simulink model "parallelParking"  (R2016b)
settings: Solver=FixedStepDiscrete  StartTime=0  StopTime=40  FixedStep=0.1  RelTol=1e-3  EnableMultiTasking=on
model workspace (MAT data in the model file):
  LANE_WIDTH = 0.5
  WORLD_SIZE = Simulink.Parameter
  WORLD_SIZE.Value = 5
  WORLD_SIZE.DataType = 'auto'
  WORLD_SIZE.Dimensions = [1 1]
  dt = Simulink.Parameter
  dt.Value = 0.05
  dt.DataType = 'auto'
  dt.Dimensions = [1 1]
values from neighbouring files (symbols this model uses):
  WORLD_SIZE = 5    [simulation.m]    (also in stateflowSim.m)
settings Model: Creator=larry  LastModifiedBy=larry
settings SolverCC: AutoInsertRateTranBlk=on
settings DataIOCC: LimitDataPoints=on
settings OptimizationCC: LifeSpan=inf
settings DebuggingCC: AllowSymbolicDim=off  SFUnexpectedBacktrackingDiag=warning  SFNoUnconditionalDefaultTransitionDiag=warning  SFExecutionAtInitializationDiag=none
settings GRTTargetCC: TargetLangStandard=C89/C90 (ANSI)  GeneratePreprocessorConditionals=Disable all
settings ConfigComp: CovMetricSettings=dw  CovHtmlReporting=on  CovSaveCumulativeToWorkspaceVar=on  CovSaveSingleToWorkspaceVar=on  CovExternalEMLEnable=off  CovSFcnEnable=off

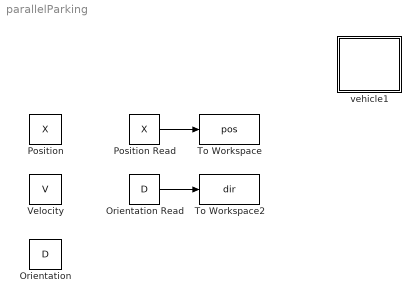
== system parallelParking ==
  Orientation : DataStoreMemory  DataStoreName=D  InitialValue=[1 1 1 1 1 1;0 0 0 0 0 0]  ShowAdditionalParam=off  OutDataTypeStr=double
  Orientation Read : DataStoreRead  DataStoreName=D
  Position : DataStoreMemory  DataStoreName=X  InitialValue="[-5 -4  -2 1 2 3; 0.25 -0.25 -0.25 -0.25 -0.25 -0.25]"  ShowAdditionalParam=off  OutDataTypeStr=double
  Position Read : DataStoreRead  DataStoreName=X
  To Workspace : ToWorkspace  VariableName=pos  SampleTime=-1
  To Workspace2 : ToWorkspace  VariableName=dir  SampleTime=-1
  Velocity : DataStoreMemory  DataStoreName=V  InitialValue=[0 0 0 0 0 0;0 0 0 0 0 0]  ShowAdditionalParam=off  OutDataTypeStr=double
  "vehicle1 " : Stateflow chart  TreatAsAtomicUnit=on
  wires:
  Position Read/1 -> To Workspace/1
  Orientation Read/1 -> To Workspace2/1

== stateflow chart parallelParking/vehicle1  ==
  state Init
    en:
    V(:,this) = V_LOW * D(:,this);
  state Straight
    state Normal
      state Acc
        en:
        a = [A_MAX; 0];
        du:
        accelerateDrive;
      state FixedRate
        du:
        fixedRateDrive;
      (default) -> Acc
      Acc -> FixedRate : [higherThan(V_LOW)]
    state Adjust
      du:
      adjustDrive;
    (default) -> Normal [order 1] : [atLaneMiddle]
    (default) -> Straight.Adjust [order 2]
    Straight.Adjust -> Normal : [atLaneMiddle]
  state FindParkingSpace
    du:
    fixedRateDrive;
  state ParallelWithFrontCar
    en:
    a = brakeToStopAt(computeStopPos());
    du:
    slowDownDrive();
  state Wait
  state Leaving
    state Right
      en:
      V(:,this) = V_PARK*D(:,this);
      dtheta = V_PARK*dt / radius;
      du:
      rightDrive;
    state Back
      en:
      V(:,this) = V_PARK*D(:,this)*(-1);
      du:
      backDrive;
    state Left
      en:
      V(:,this) = V_PARK*D(:,this);
      dtheta = (-1)*V_PARK*dt / radius;
      du:
      leftDrive;
    state Forward
      du:
      fixedRateDrive;
    (default) -> Leaving.Back
    Leaving.Back -> Left : [reachBack]
    Forward -> Right : [rWheelReachLine]
    Left -> Forward : [enoughAngle]
  state Parking
    state BackRight
      en:
      V(:,this) = V_PARK*D(:,this)*(-1);
      dtheta = V_PARK*dt / radius;
      du:
      backRightDrive;
    state Adjust
      en:
      V(:,this) = V_PARK*D(:,this);
      du:
      fixedRateDrive;
    state BackLeft
      en:
      V(:,this) = V_PARK*D(:,this)*(-1);
      dtheta = (-1) * V_PARK*dt / radius;
      du:
      backLeftDrive;
    state Back
      en:
      V(:,this) = V_PARK*D(:,this)*(-1);
      du:
      backDrive;
    (default) -> BackRight
    BackLeft -> Parking.Adjust : [parallelWithLane]
    BackRight -> Parking.Back : [rWheelReachLine]
    Parking.Back -> BackLeft : [lWheelReachLine]
  state Parked
  (default) -> Init
  Init -> FindParkingSpace
  FindParkingSpace -> ParallelWithFrontCar : [hasParkingSpace]
  ParallelWithFrontCar -> Wait : [isStopped]
  Leaving -> Straight : [in(Leaving.Right) && ...
      |  parallelWithLane]
  Wait -> Parking : after(1, sec)
  Parked -> Leaving : after(2, sec)
  Parking -> Parked : [in(Parking.Adjust) && ...
      | parkedCenter]
  data: res function_output; target function_input; res function_output; res function_output; res function_output; res function_output; pos function_input; res function_output; res function_output; res function_output; res function_output; res function_output; res function_output; res function_output; res function_output; X data_store_memory; D data_store_memory; V_LOW constant double =1; a local double size=[2 1] =[0; 0]; this local uint8 size=1 =uint8(1); V data_store_memory; V_MIN constant double =0.125; WORLD_SIZE parameter; dt parameter; radius local =0.5; dtheta local; PARK_DELTA constant double =0.125; EPS constant double =0.01; V_PARK constant double =0.4; LATERAL_DX constant double =0.0009765625; A_MAX constant double =2.5
  function res = higherThan(target):
    | function res = higherThan(target)
    | 
    | v_norm = norm(V(:,this));
    | 
    | res = (v_norm >= target) || ((target - norm(V(:,this))) < V_MIN);
  function accelerateDrive:
    | function accelerateDrive
    | 
    | x = X(:,this);
    | v = V(:,this);
    | a = D(:,this) * A_MAX;
    | 
    | x = x + v * dt + 0.5 * a * dt * dt;
    | v = v + a * dt;
    | 
    | % a rounded world
    | if x(1) > WORLD_SIZE
    |     x(1) = -WORLD_SIZE;
    | elseif x(1) < -WORLD_SIZE
    |     x(1) = WORLD_SIZE;
    | elseif x(2) > WORLD_SIZE
    |     x(2) = -WORLD_SIZE;
    | elseif x(2) < -WORLD_SIZE
    |     x(2) = WORLD_SIZE;
    | end
    | 
    | X(:,this) = x;
    | V(:,this) = v;
  function slowDownDrive:
    | function slowDownDrive
    | 
    | x = X(:,this);
    | v = V(:,this);
    | d = D(:, this);
    | v_norm = norm(v);
    | 
    | 
    | if v_norm <= V_MIN && (dot(a, d) <= 0)
    |     v = 0 * D(:,this);
    |     a = 0 * D(:,this);
    |     return;
    | end
    | 
    | x = x + v * dt + 0.5 * a * dt * dt;
    | v = v + a * dt;
    | 
    | % a rounded world
    | if x(1) > WORLD_SIZE
    |     x(1) = -WORLD_SIZE;
    | elseif x(1) < -WORLD_SIZE
    |     x(1) = WORLD_SIZE;
    | elseif x(2) > WORLD_SIZE
    |     x(2) = -WORLD_SIZE;
    | elseif x(2) < -WORLD_SIZE
    |     x(2) = WORLD_SIZE;
    | end
    | 
    | X(:,this) = x;
    | V(:,this) = v;
  function fixedRateDrive:
    | function fixedRateDrive
    |  
    | x = X(:,this);
    | v = V(:,this);
    | 
    | % update new position
    | x = x + v * dt;
    | 
    | % a rounded world
    | if x(1) > WORLD_SIZE
    |     x(1) = -WORLD_SIZE;
    | elseif x(1) < -WORLD_SIZE
    |     x(1) = WORLD_SIZE;
    | elseif x(2) > WORLD_SIZE
    |     x(2) = -WORLD_SIZE;
    | elseif x(2) < -WORLD_SIZE
    |     x(2) = WORLD_SIZE;
    | end
    | 
    | X(:,this) = x;
  function res = hasParkingSpace:
    | function res = hasParkingSpace
    | 
    | RANGE = 2 * WORLD_SIZE;
    | 
    | x = X(:,this);
    | 
    | i = x(1);
    | ii = X(1,:);
    | diff = mod((ii - i + RANGE), RANGE);
    | 
    | res = isempty(find((diff > 0 & diff <= 1), 1));
  function backRightDrive:
    | function backRightDrive
    |  
    | % right turn radius is larger than zero
    | 
    | x = X(:,this);
    | v = V(:,this);
    | d = D(:,this);
    | 
    | rot = [cos(dtheta) -sin(dtheta); sin(dtheta) cos(dtheta)];
    | % rot1 = [cos(dtheta) sin(dtheta); -sin(dtheta) cos(dtheta)];
    | 
    | hdtheta = abs(dtheta)/2;
    | % the following theta is always positive
    | dx1 = radius * sin(hdtheta) * (-d);
    | 
    | v = rot * v;
    | d = rot * d;
    | 
    | dx2 = radius * sin(hdtheta) * (-d);
    | x = x + dx1 + dx2;
    | 
    | X(:,this) = x;
    | V(:,this) = v;
    | D(:,this) = d;
  function res = rWheelReachLine:
    | function res = rWheelReachLine
    | 
    | x = X(:,this);
    | d = D(:,this);
    | 
    | rot = [4/5 -3/5; 3/5 4/5];
    | 
    | delta = rot * d * (-1) * 0.25;
    | rb = x + delta;
    | 
    | res = abs((0 - PARK_DELTA) - rb(2)) < EPS;
  function res = lWheelReachLine:
    | function res = lWheelReachLine
    |  
    | x = X(:,this);
    | d = D(:,this);
    | 
    | rot = [4/5 3/5; -3/5 4/5];
    | 
    | delta = rot * d * (-1) * 0.25;
    | rb = x + delta;
    | 
    | res = abs((0 - PARK_DELTA) - rb(2)) < EPS;
  function backDrive:
    | function backDrive
    |  
    | x = X(:,this);
    | v = V(:,this);
    | d = D(:,this);
    | 
    | if dot(v, d) >= 0
    |     v = V_MIN * (-1) * D(:,this);
    |     V(:,this) = v;
    | end
    | 
    | x = x + v * dt;
    | 
    | X(:,this) = x;
  function backLeftDrive:
    | function backLeftDrive
    |  
    | % dtheta of left turn must be negative
    | 
    | x = X(:,this);
    | v = V(:,this);
    | d = D(:,this);
    | 
    | rot = [cos(dtheta) -sin(dtheta); sin(dtheta) cos(dtheta)];
    | % rot1 = [cos(dtheta) sin(dtheta); -sin(dtheta) cos(dtheta)];
    | 
    | hdtheta = abs(dtheta)/2;
    | % the following theta is always positive
    | dx1 = radius * sin(hdtheta) * (-d);
    | 
    | v = rot * v;
    | d = rot * d;
    | 
    | dx2 = radius * sin(hdtheta) * (-d);
    | x = x + dx1 + dx2;
    | 
    | X(:,this) = x;
    | V(:,this) = v;
    | D(:,this) = d;
  function res = parallelWithLane:
    | function res = parallelWithLane
    | 
    | d = D(:,this);
    | lane = [1; 0];
    | 
    | res = dot(lane, d) >= 0.99999;
  function res = brakeToStopAt(pos):
    | function res = brakeToStopAt(pos)
    | 
    | res = [0; 0];
    | 
    | x = X(:,this);
    | v = V(:,this);
    | d = D(:,this);
    | 
    | dist = norm(pos - x);
    |  
    | vnorm = norm(v);
    | res = (-1)*d*vnorm*vnorm/2/dist;
  function res = computeStopPos:
    | function res = computeStopPos
    | 
    | x = X(:, this);
    | 
    | % V(:, this) = 0 * D(:, this);
    | % res = x;
    | 
    | pos = floor(x(1))+1;
    | next = pos + 1;
    | 
    | ii = X(1,:);
    | assert(isempty(find(ii == pos, 1)), 'should not have a car there');
    | 
    | res = [next - 0.5 + (0.4)/2; x(2)];
    | % small = isempty(find(ii == next, 1));
  function res = parkedCenter:
    | function res = parkedCenter
    | 
    | x = X(:,this);
    | 
    | target = round(x(1));
    | res = abs(x(1)-target) < EPS;
  function res = isStopped:
    | function res = isStopped
    | 
    | res = (norm(V(:,this)) < V_MIN);
  function rightDrive:
    | function rightDrive
    |  
    | % dtheta of left turn must be negative
    | 
    | x = X(:,this);
    | v = V(:,this);
    | d = D(:,this);
    | 
    | rot = [cos(dtheta) sin(dtheta); -sin(dtheta) cos(dtheta)];
    | 
    | % the following theta is always positive
    | hdtheta = abs(dtheta)/2;
    | dx1 = radius * sin(hdtheta) * d;
    | 
    | v = rot * v;
    | d = rot * d;
    | 
    | dx2 = radius * sin(hdtheta) * d;
    | x = x + dx1 + dx2;
    | 
    | X(:,this) = x;
    | V(:,this) = v;
    | D(:,this) = d;
  function leftDrive:
    | function leftDrive
    |  
    | % dtheta of left turn must be negative
    | 
    | x = X(:,this);
    | v = V(:,this);
    | d = D(:,this);
    | 
    | rot = [cos(dtheta) sin(dtheta); -sin(dtheta) cos(dtheta)];
    | 
    | % the following theta is always positive
    | hdtheta = abs(dtheta)/2;
    | dx1 = radius * sin(hdtheta) * d;
    | 
    | v = rot * v;
    | d = rot * d;
    | 
    | dx2 = radius * sin(hdtheta) * d;
    | x = x + dx1 + dx2;
    | 
    | X(:,this) = x;
    | V(:,this) = v;
    | D(:,this) = d;
  function res = reachBack:
    | function res = reachBack
    |  
    | x = X(:,this);
    | 
    | target = (round(x(1))-0.5)+0.2;
    | res = abs(x(1)-target) < EPS;
  function res = alwaysFalse:
    | function res = alwaysFalse
    |  
    | res = false;
  function res = enoughAngle:
    | function res = enoughAngle
    |  
    | d = D(:,this);
    | lane = [1; 0];
    | 
    | val = cos(deg2rad(30));
    | 
    | res = (dot(d, lane) - val) < EPS;
  function res = atLaneMiddle:
    | function res = atLaneMiddle
    |  
    | x = X(:,this);
    | 
    | res = (x(2) - floor(x(2))) == 0.25;
  function adjustDrive:
    | function adjustDrive
    |  
    | x = X(:,this);
    | v = V(:,this);
    | 
    | dx = 0.25 - x(2);
    | 
    | if dx >= 0
    |     dx = min(LATERAL_DX, dx);
    | else
    |     dx = max(-LATERAL_DX, dx);
    | end
    | 
    | x = x + [0; dx] + v * dt;
    | 
    | X(:,this) = x;
